simulink model "PV_Model3"  (R2017a)
settings: Solver=VariableStepAuto  StartTime=0.0  StopTime=0.0001  MaxStep=1e-4  RelTol=1e-3
values from neighbouring files (symbols this model uses):
  Eg0 = 1.1    [PV_Model_Parameters.m]    (also in Simulation.m)
  Irr = 900    [PV_Model_Parameters.m]
  Isc = 6.11    [PV_Model_Parameters.m]    (also in Simulation.m)
  K = 1.3805e-23    [PV_Model_Parameters.m]    (also in Simulation.m)
  ki = 0.002    [PV_Model_Parameters.m]    (also in Simulation.m)
  n = 1.2    [PV_Model_Parameters.m]    (also in Simulation.m)
  Np = 1    [PV_Model_Parameters.m]    (also in Simulation.m)
  Ns = 36    [PV_Model_Parameters.m]    (also in Simulation.m)
  q = 1.6e-19    [PV_Model_Parameters.m]    (also in Simulation.m)
  Rs = 0.0001    [PV_Model_Parameters.m]    (also in Simulation.m)
  Rsh = 1000    [PV_Model_Parameters.m]    (also in Simulation.m)
  T2M = 30    [PV_Model_Parameters.m]
  Tn = 298.15    [PV_Model_Parameters.m]    (also in Simulation.m)
  Voc = 21.6    [PV_Model_Parameters.m]    (also in Simulation.m)
libraries: powerlib x6
settings Model: Creator=idpdl  LastModifiedBy=idpdl

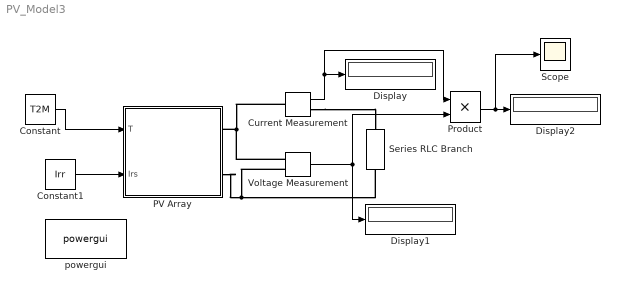
== system PV_Model3 ==
  Constant : Constant  Value=T2M
  Constant1 : Constant  Value=Irr
  Current Measurement : powerlib/Measurements/Current Measurement  PhasorSimulation=off  OutputType=Complex  PSBequivalent=0
  Display : Display
  Display1 : Display
  Display2 : Display
  PV Array : Subsystem
  Product : Product
  Scope : Scope
  Series RLC Branch : powerlib/Elements/Series RLC Branch  LConnTagsString=__new0  RConnTagsString=__new0  BranchType=R  Resistance=3.1  Inductance=1e-3  SetiL0=off  InitialCurrent=0  Capacitance=1e-6  Setx0=off  InitialVoltage=0  Measurements=None
  Voltage Measurement : powerlib/Measurements/Voltage Measurement  PhasorSimulation=off  OutputType=Complex  PSBequivalent=0
  powergui : powerlib/powergui  Priority=1  SimulationMode=Continuous  SampleTime=50e-6  frequency=60  Iterations=50  frequencyindice=0  Pbase=100e6  ErrMax=1e-4  UnitsV=kV  UnitsW=MW  buscounter=0  FunctionMessages=off  echomessages=off  EnableUseOfTLC=off  CurrentSourceSwitches=off  DisableSnubberDevices=off  DisableRonSwitches=off  DisableVfSwitches=off  DisplayEquations=off  SolverType=Tustin/Backward Euler (TBE)  Interpol=off  ExternalGateDelay=off  methode=off  Ts=100  x0status=blocks  SPID=on  SwTol=0  HookPort=off  RestoreLinks=warning  ResistiveCurrentMeasurement=off  Frange=[0:2:500]  Ylog=off  Xlog=on  ShowGrid=off  save=off  variable=ZData  structure=0  ZoomFFT=off  StartTime=0.0  cycles=1  DisplayStyle=1  fundamental=60  FreqAxis=off  MaxFrequency=1000  frequencyindicesteady=1  RmsSteady=1  display=off
  wires:
  Constant/1 -> PV Array/1(T)
  Constant1/1 -> PV Array/2(Irs)
  Current Measurement/1 -> Display/1, Product/1
  Voltage Measurement/1 -> Display1/1, Product/2
  Product/1 -> Scope/1, Display2/1
  connections:
  PV Array/RConn2 -- Voltage Measurement/LConn2 -- Series RLC Branch/LConn1
  Current Measurement/LConn1 -- Voltage Measurement/LConn1 -- PV Array/RConn1
  Current Measurement/RConn1 -- Series RLC Branch/RConn1

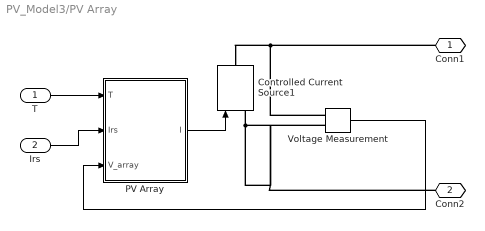
== system PV_Model3/PV Array ==
  T : Inport
  Irs : Inport  Port=2
  Controlled Current Source1 : powerlib/Electrical Sources/Controlled Current Source  Initialize=on  Source_Type=DC  Amplitude=0  Phase=0  Frequency=0  Measurements=None
  PV Array : Subsystem
  Voltage Measurement : powerlib/Measurements/Voltage Measurement  PhasorSimulation=off  OutputType=Complex  PSBequivalent=0
  Conn1 : PMIOPort  Port=1  Side=Right
  Conn2 : PMIOPort  Port=2  Side=Right
  wires:
  Voltage Measurement/1 -> PV Array/3(V_array)
  PV Array/1(I) -> Controlled Current Source1/1
  T/1 -> PV Array/1(T)
  Irs/1 -> PV Array/2(Irs)
  connections:
  Controlled Current Source1/LConn1 -- Conn2/RConn1 -- Voltage Measurement/LConn2
  Voltage Measurement/LConn1 -- Conn1/RConn1 -- Controlled Current Source1/RConn1

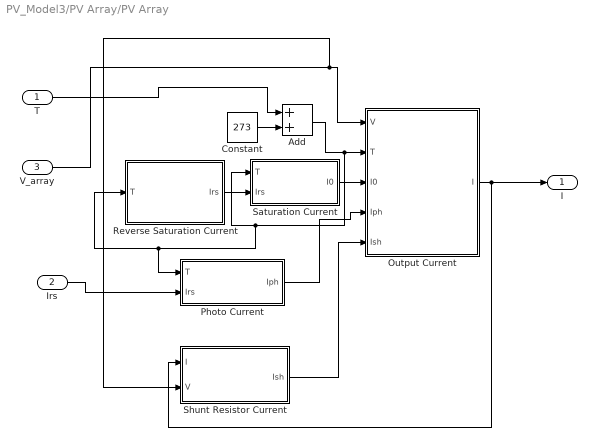
== system PV_Model3/PV Array/PV Array ==
  T : Inport
  Irs : Inport  Port=2
  V_array : Inport  Port=3
  Add : Sum
  Constant : Constant  Value=273
  Output Current : Subsystem
  Photo Current : Subsystem
  Reverse Saturation Current : Subsystem
  Saturation Current : Subsystem
  Shunt Resistor Current : Subsystem
  I : Outport
  wires:
  T/1 -> Add/1
  Shunt Resistor Current/1(Ish) -> Output Current/5(Ish)
  Constant/1 -> Add/2
  Photo Current/1(Iph) -> Output Current/4(Iph)
  Irs/1 -> Photo Current/2(Irs)
  Add/1 -> Photo Current/1(T), Reverse Saturation Current/1(T), Saturation Current/1(T), Output Current/2(T)
  Output Current/1(I) -> I/1, Shunt Resistor Current/1(I)
  Reverse Saturation Current/1(Irs) -> Saturation Current/2(Irs)
  Saturation Current/1(I0) -> Output Current/3(I0)
  V_array/1 -> Shunt Resistor Current/2(V), Output Current/1(V)

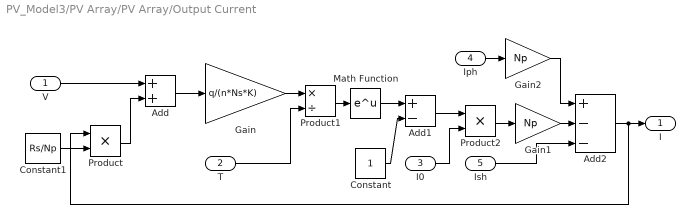
== system PV_Model3/PV Array/PV Array/Output Current ==
  V : Inport
  T : Inport  Port=2
  I0 : Inport  Port=3
  Iph : Inport  Port=4
  Ish : Inport  Port=5
  Add : Sum
  Add1 : Sum  Inputs=+-
  Add2 : Sum  Inputs=+--
  Constant : Constant
  Constant1 : Constant  Value=Rs/Np
  Gain : Gain  Gain=q/(n*Ns*K)
  Gain1 : Gain  Gain=Np
  Gain2 : Gain  Gain=Np
  Math Function : Math  SaturateOnIntegerOverflow=on
  Product : Product
  Product1 : Product  Inputs=*/
  Product2 : Product
  I : Outport
  wires:
  Product/1 -> Add/2
  Constant1/1 -> Product/2
  Add/1 -> Gain/1
  Gain/1 -> Product1/1
  T/1 -> Product1/2
  Constant/1 -> Add1/2
  Product1/1 -> Math Function/1
  Math Function/1 -> Add1/1
  Add1/1 -> Product2/1
  I0/1 -> Product2/2
  Iph/1 -> Gain2/1
  Ish/1 -> Add2/3
  Add2/1 -> Product/1, I/1
  V/1 -> Add/1
  Gain1/1 -> Add2/2
  Product2/1 -> Gain1/1
  Gain2/1 -> Add2/1

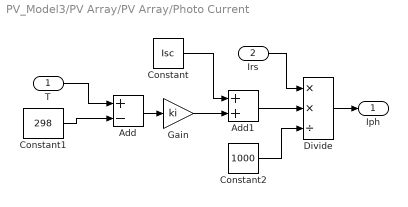
== system PV_Model3/PV Array/PV Array/Photo Current ==
  T : Inport
  Irs : Inport  Port=2
  Add : Sum  Inputs=+-
  Add1 : Sum
  Constant : Constant  Value=Isc
  Constant1 : Constant  Value=298
  Constant2 : Constant  Value=1000
  Divide : Product  Inputs=**/
  Gain : Gain  Gain=ki
  Iph : Outport
  wires:
  T/1 -> Add/1
  Constant1/1 -> Add/2
  Add/1 -> Gain/1
  Constant/1 -> Add1/1
  Gain/1 -> Add1/2
  Add1/1 -> Divide/2
  Irs/1 -> Divide/1
  Constant2/1 -> Divide/3
  Divide/1 -> Iph/1

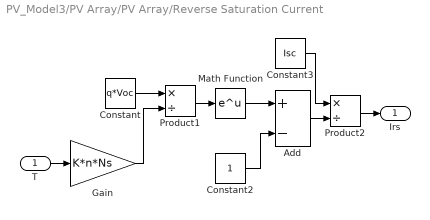
== system PV_Model3/PV Array/PV Array/Reverse Saturation Current ==
  T : Inport
  Add : Sum  Inputs=+-
  Constant : Constant  Value=q*Voc
  Constant2 : Constant
  Constant3 : Constant  Value=Isc
  Gain : Gain  Gain=K*n*Ns
  Math Function : Math  SaturateOnIntegerOverflow=on
  Product1 : Product  Inputs=*/
  Product2 : Product  Inputs=*/
  Irs : Outport
  wires:
  T/1 -> Gain/1
  Constant/1 -> Product1/1
  Gain/1 -> Product1/2
  Product1/1 -> Math Function/1
  Math Function/1 -> Add/1
  Constant2/1 -> Add/2
  Constant3/1 -> Product2/1
  Add/1 -> Product2/2
  Product2/1 -> Irs/1

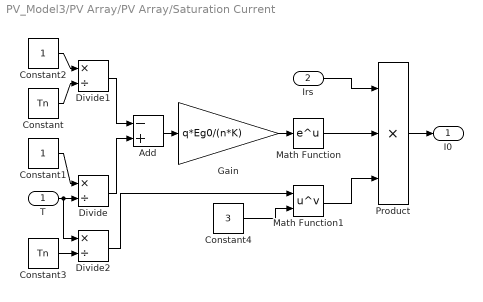
== system PV_Model3/PV Array/PV Array/Saturation Current ==
  T : Inport
  Irs : Inport  Port=2
  Add : Sum  Inputs=-+
  Constant : Constant  Value=Tn
  Constant1 : Constant
  Constant2 : Constant
  Constant3 : Constant  Value=Tn
  Constant4 : Constant  Value=3
  Divide : Product  Inputs=*/
  Divide1 : Product  Inputs=*/
  Divide2 : Product  Inputs=*/
  Gain : Gain  Gain=q*Eg0/(n*K)
  Math Function : Math  SaturateOnIntegerOverflow=on
  Math Function1 : Math  Operator=pow  SaturateOnIntegerOverflow=on
  Product : Product  Inputs=3
  I0 : Outport
  wires:
  Constant1/1 -> Divide/1
  T/1 -> Divide2/1, Divide/2
  Constant2/1 -> Divide1/1
  Constant/1 -> Divide1/2
  Divide1/1 -> Add/1
  Divide/1 -> Add/2
  Add/1 -> Gain/1
  Gain/1 -> Math Function/1
  Constant3/1 -> Divide2/2
  Divide2/1 -> Math Function1/1
  Constant4/1 -> Math Function1/2
  Math Function/1 -> Product/2
  Math Function1/1 -> Product/3
  Irs/1 -> Product/1
  Product/1 -> I0/1

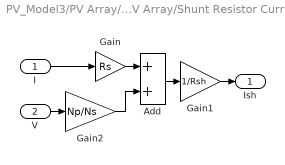
== system PV_Model3/PV Array/PV Array/Shunt Resistor Current ==
  I : Inport
  V : Inport  Port=2
  Add : Sum
  Gain : Gain  Gain=Rs
  Gain1 : Gain  Gain=1/Rsh
  Gain2 : Gain  Gain=Np/Ns
  Ish : Outport
  wires:
  I/1 -> Gain/1
  Gain/1 -> Add/1
  Add/1 -> Gain1/1
  Gain1/1 -> Ish/1
  V/1 -> Gain2/1
  Gain2/1 -> Add/2
